simulink model "filtros_r2015b"  (R2015b)
settings: Solver=VariableStepAuto  SolverMode=SingleTasking  StartTime=0.0  StopTime=10.0  RelTol=1e-3
libraries: dsparch4 x4
(part 4 of 5)

== system filtros_r2015b/filtro_bs_iir_direct2_sos_40_fb ==
  In : Inport
  Input Quantizer : DataTypeConversion  OutDataTypeStr=fixdt(1,16,15)  RndMeth=Round  SaturateOnIntegerOverflow=on
  filter : dsparch4/Biquad Filter  FilterSource=Specify via dialog  CoeffSource=Specify via dialog  FilterObject=BQF  IIRFiltStruct=Direct form II  BiQuadCoeffs=[1 -1.11152954346655419 1.05088219447620013 1 -0.813428281179642165 0.552005579906472033;1 -1.07211536629555804 1.06865251897541036 1 -0.742197661664668717 0.854865767395351028;1 -1.0032399136855954 0.935758131903575485 1 -1.18020037227255226 0.875550994084790757;1 -1.01063368621325411 1.03083232416279569 1 -0.8635074436780521 0.959930995951585597;1 -1.05770999558857559 0.951581007807177359 1 -1.17581613832315401 0.964163580544992183;1 -0.980405596804986956 0.97009053687980229 1 -0.90563072038096426 0.990340187952881257;1 -1.1019651730511173 0.999999494703609493 1 -1.16875024700793517 0.991207917022611129]  ScaleValues=[0.619240669533610344;1;1;1;1;1;1;1]  IC=0  ICnum=0  ICden=0  a0Flag=Warning  optimizeScaleValues=on  ScaleValueMode=Specify via input port (g)  InputProcessing=Columns as channels (frame based)  roundingMode=Convergent  overflowMode=off  stageInputMode=Binary point scaling  stageInputWordLength=16  stageInputFracLength=10  stageOutputMode=Binary point scaling  stageOutputWordLength=16  stageOutputFracLength=11  firstCoeffMode=Binary point scaling  firstCoeffWordLength=40  firstCoeffFracLength=38  scaleValueFracLength=39  prodOutputMode=Binary point scaling  prodOutputWordLength=56  prodOutputFracLength=53  denProdOutputFracLength=53  accumMode=Binary point scaling  accumWordLength=40  accumFracLength=35  denAccumFracLength=35  memoryMode=Binary point scaling  memoryWordLength=16  memoryFracLength=15  secondMemoryFracLength=15  outputMode=Binary point scaling  outputWordLength=16  outputFracLength=11
  Out : Outport
  wires:
  In/1 -> Input Quantizer/1
  Input Quantizer/1 -> filter/1
  filter/1 -> Out/1

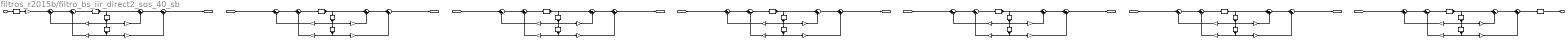
== system filtros_r2015b/filtro_bs_iir_direct2_sos_40_sb ==
  Input : Inport
  CastState{1..7} (7 alike) : DataTypeConversion  OutDataTypeStr=fixdt(1,16,15)  RndMeth=Convergent
  ConvertIn : DataTypeConversion  OutDataTypeStr=fixdt(1,16,15)  RndMeth=Nearest  SaturateOnIntegerOverflow=on
  ConvertOut : DataTypeConversion  OutDataTypeStr=fixdt(1,16,11)  RndMeth=Convergent
  Delay{11..17,21..27} (14 alike) : Delay  DelayLength=1  InitialCondition=0
  SumA{21..27,31..37} (14 alike) : Sum  Inputs=|+-  AccumDataTypeStr=fixdt(1,40,35)  OutDataTypeStr=fixdt(1,40,35)  RndMeth=Convergent
  SumB{21..27,31..37} (14 alike) : Sum  Inputs=|++  AccumDataTypeStr=fixdt(1,40,35)  OutDataTypeStr=fixdt(1,40,35)  RndMeth=Convergent
  a(2)(1) : Gain  Gain=-0.813428281179642165  ParamDataTypeStr=fixdt(1,40,38)  OutDataTypeStr=fixdt(1,56,53)  RndMeth=Convergent
  a(2)(2) : Gain  Gain=-0.742197661664668717  ParamDataTypeStr=fixdt(1,40,38)  OutDataTypeStr=fixdt(1,56,53)  RndMeth=Convergent
  a(2)(3) : Gain  Gain=-1.18020037227255226  ParamDataTypeStr=fixdt(1,40,38)  OutDataTypeStr=fixdt(1,56,53)  RndMeth=Convergent
  a(2)(4) : Gain  Gain=-0.8635074436780521  ParamDataTypeStr=fixdt(1,40,38)  OutDataTypeStr=fixdt(1,56,53)  RndMeth=Convergent
  a(2)(5) : Gain  Gain=-1.17581613832315401  ParamDataTypeStr=fixdt(1,40,38)  OutDataTypeStr=fixdt(1,56,53)  RndMeth=Convergent
  a(2)(6) : Gain  Gain=-0.90563072038096426  ParamDataTypeStr=fixdt(1,40,38)  OutDataTypeStr=fixdt(1,56,53)  RndMeth=Convergent
  a(2)(7) : Gain  Gain=-1.16875024700793517  ParamDataTypeStr=fixdt(1,40,38)  OutDataTypeStr=fixdt(1,56,53)  RndMeth=Convergent
  a(3)(1) : Gain  Gain=0.552005579906472033  ParamDataTypeStr=fixdt(1,40,38)  OutDataTypeStr=fixdt(1,56,53)  RndMeth=Convergent
  a(3)(2) : Gain  Gain=0.854865767395351028  ParamDataTypeStr=fixdt(1,40,38)  OutDataTypeStr=fixdt(1,56,53)  RndMeth=Convergent
  a(3)(3) : Gain  Gain=0.875550994084790757  ParamDataTypeStr=fixdt(1,40,38)  OutDataTypeStr=fixdt(1,56,53)  RndMeth=Convergent
  a(3)(4) : Gain  Gain=0.959930995951585597  ParamDataTypeStr=fixdt(1,40,38)  OutDataTypeStr=fixdt(1,56,53)  RndMeth=Convergent
  a(3)(5) : Gain  Gain=0.964163580544992183  ParamDataTypeStr=fixdt(1,40,38)  OutDataTypeStr=fixdt(1,56,53)  RndMeth=Convergent
  a(3)(6) : Gain  Gain=0.990340187952881257  ParamDataTypeStr=fixdt(1,40,38)  OutDataTypeStr=fixdt(1,56,53)  RndMeth=Convergent
  a(3)(7) : Gain  Gain=0.991207917022611129  ParamDataTypeStr=fixdt(1,40,38)  OutDataTypeStr=fixdt(1,56,53)  RndMeth=Convergent
  b(2)(1) : Gain  Gain=-1.11152954346655419  ParamDataTypeStr=fixdt(1,40,38)  OutDataTypeStr=fixdt(1,56,53)  RndMeth=Convergent
  b(2)(2) : Gain  Gain=-1.07211536629555804  ParamDataTypeStr=fixdt(1,40,38)  OutDataTypeStr=fixdt(1,56,53)  RndMeth=Convergent
  b(2)(3) : Gain  Gain=-1.0032399136855954  ParamDataTypeStr=fixdt(1,40,38)  OutDataTypeStr=fixdt(1,56,53)  RndMeth=Convergent
  b(2)(4) : Gain  Gain=-1.01063368621325411  ParamDataTypeStr=fixdt(1,40,38)  OutDataTypeStr=fixdt(1,56,53)  RndMeth=Convergent
  b(2)(5) : Gain  Gain=-1.05770999558857559  ParamDataTypeStr=fixdt(1,40,38)  OutDataTypeStr=fixdt(1,56,53)  RndMeth=Convergent
  b(2)(6) : Gain  Gain=-0.980405596804986956  ParamDataTypeStr=fixdt(1,40,38)  OutDataTypeStr=fixdt(1,56,53)  RndMeth=Convergent
  b(2)(7) : Gain  Gain=-1.1019651730511173  ParamDataTypeStr=fixdt(1,40,38)  OutDataTypeStr=fixdt(1,56,53)  RndMeth=Convergent
  b(3)(1) : Gain  Gain=1.05088219447620013  ParamDataTypeStr=fixdt(1,40,38)  OutDataTypeStr=fixdt(1,56,53)  RndMeth=Convergent
  b(3)(2) : Gain  Gain=1.06865251897541036  ParamDataTypeStr=fixdt(1,40,38)  OutDataTypeStr=fixdt(1,56,53)  RndMeth=Convergent
  b(3)(3) : Gain  Gain=0.935758131903575485  ParamDataTypeStr=fixdt(1,40,38)  OutDataTypeStr=fixdt(1,56,53)  RndMeth=Convergent
  b(3)(4) : Gain  Gain=1.03083232416279569  ParamDataTypeStr=fixdt(1,40,38)  OutDataTypeStr=fixdt(1,56,53)  RndMeth=Convergent
  b(3)(5) : Gain  Gain=0.951581007807177359  ParamDataTypeStr=fixdt(1,40,38)  OutDataTypeStr=fixdt(1,56,53)  RndMeth=Convergent
  b(3)(6) : Gain  Gain=0.97009053687980229  ParamDataTypeStr=fixdt(1,40,38)  OutDataTypeStr=fixdt(1,56,53)  RndMeth=Convergent
  b(3)(7) : Gain  Gain=0.999999494703609493  ParamDataTypeStr=fixdt(1,40,38)  OutDataTypeStr=fixdt(1,56,53)  RndMeth=Convergent
  s(1) : Gain  Gain=0.619240669533610344  ParamDataTypeStr=fixdt(1,40,39)  OutDataTypeStr=fixdt(1,16,10)  RndMeth=Convergent
  Output : Outport
  wires:
  Input/1 -> ConvertIn/1
  s(1)/1 -> SumA21/1
  SumA21/1 -> SumA31/1
  SumA31/1 -> CastState1/1
  CastState1/1 -> SumB21/1, Delay11/1
  SumB21/1 -> SumB31/1
  SumB31/1 -> [Sect1]
  a(2)(1)/1 -> SumA21/2
  Delay11/1 -> a(2)(1)/1, b(2)(1)/1, Delay21/1
  b(2)(1)/1 -> SumB21/2
  a(3)(1)/1 -> SumA31/2
  Delay21/1 -> a(3)(1)/1, b(3)(1)/1
  b(3)(1)/1 -> SumB31/2
  ConvertIn/1 -> s(1)/1
  [Sect1] -> SumA22/1
  SumA22/1 -> SumA32/1
  SumA32/1 -> CastState2/1
  CastState2/1 -> SumB22/1, Delay12/1
  SumB22/1 -> SumB32/1
  SumB32/1 -> [Sect2]
  a(2)(2)/1 -> SumA22/2
  Delay12/1 -> a(2)(2)/1, b(2)(2)/1, Delay22/1
  b(2)(2)/1 -> SumB22/2
  a(3)(2)/1 -> SumA32/2
  Delay22/1 -> a(3)(2)/1, b(3)(2)/1
  b(3)(2)/1 -> SumB32/2
  [Sect2] -> SumA23/1
  SumA23/1 -> SumA33/1
  SumA33/1 -> CastState3/1
  CastState3/1 -> SumB23/1, Delay13/1
  SumB23/1 -> SumB33/1
  SumB33/1 -> [Sect3]
  a(2)(3)/1 -> SumA23/2
  Delay13/1 -> a(2)(3)/1, b(2)(3)/1, Delay23/1
  b(2)(3)/1 -> SumB23/2
  a(3)(3)/1 -> SumA33/2
  Delay23/1 -> a(3)(3)/1, b(3)(3)/1
  b(3)(3)/1 -> SumB33/2
  [Sect3] -> SumA24/1
  SumA24/1 -> SumA34/1
  SumA34/1 -> CastState4/1
  CastState4/1 -> SumB24/1, Delay14/1
  SumB24/1 -> SumB34/1
  SumB34/1 -> [Sect4]
  a(2)(4)/1 -> SumA24/2
  Delay14/1 -> a(2)(4)/1, b(2)(4)/1, Delay24/1
  b(2)(4)/1 -> SumB24/2
  a(3)(4)/1 -> SumA34/2
  Delay24/1 -> a(3)(4)/1, b(3)(4)/1
  b(3)(4)/1 -> SumB34/2
  [Sect4] -> SumA25/1
  SumA25/1 -> SumA35/1
  SumA35/1 -> CastState5/1
  CastState5/1 -> SumB25/1, Delay15/1
  SumB25/1 -> SumB35/1
  SumB35/1 -> [Sect5]
  a(2)(5)/1 -> SumA25/2
  Delay15/1 -> a(2)(5)/1, b(2)(5)/1, Delay25/1
  b(2)(5)/1 -> SumB25/2
  a(3)(5)/1 -> SumA35/2
  Delay25/1 -> a(3)(5)/1, b(3)(5)/1
  b(3)(5)/1 -> SumB35/2
  [Sect5] -> SumA26/1
  SumA26/1 -> SumA36/1
  SumA36/1 -> CastState6/1
  CastState6/1 -> SumB26/1, Delay16/1
  SumB26/1 -> SumB36/1
  SumB36/1 -> [Sect6]
  a(2)(6)/1 -> SumA26/2
  Delay16/1 -> a(2)(6)/1, b(2)(6)/1, Delay26/1
  b(2)(6)/1 -> SumB26/2
  a(3)(6)/1 -> SumA36/2
  Delay26/1 -> a(3)(6)/1, b(3)(6)/1
  b(3)(6)/1 -> SumB36/2
  [Sect6] -> SumA27/1
  SumA27/1 -> SumA37/1
  SumA37/1 -> CastState7/1
  CastState7/1 -> SumB27/1, Delay17/1
  SumB27/1 -> SumB37/1
  SumB37/1 -> ConvertOut/1
  a(2)(7)/1 -> SumA27/2
  Delay17/1 -> a(2)(7)/1, b(2)(7)/1, Delay27/1
  b(2)(7)/1 -> SumB27/2
  a(3)(7)/1 -> SumA37/2
  Delay27/1 -> a(3)(7)/1, b(3)(7)/1
  b(3)(7)/1 -> SumB37/2
  ConvertOut/1 -> Output/1

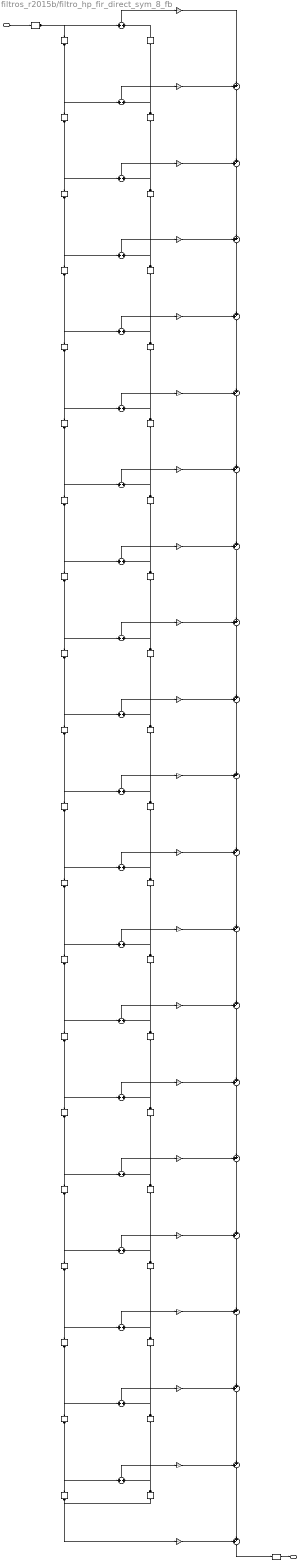
== system filtros_r2015b/filtro_hp_fir_direct_sym_8_fb ==
  Input : Inport
  BodyDelayL{2..20} (19 alike) : Delay  DelayLength=1  InitialCondition=0  InputProcessing=Columns as channels (frame based)
  BodyDelayR{2..20} (19 alike) : Delay  DelayLength=1  InitialCondition=0  InputProcessing=Columns as channels (frame based)
  BodySumL{2..20} (19 alike) : Sum  Inputs=+|+  AccumDataTypeStr=fixdt(1,17,15)  OutDataTypeStr=fixdt(1,17,15)  RndMeth=Convergent
  BodySumR{2..20} (19 alike) : Sum  Inputs=++|  AccumDataTypeStr=fixdt(1,26,24)  OutDataTypeStr=fixdt(1,26,24)  RndMeth=Convergent
  ConvertIn : DataTypeConversion  OutDataTypeStr=fixdt(1,16,15)  RndMeth=Nearest  SaturateOnIntegerOverflow=on
  ConvertOut : DataTypeConversion  OutDataTypeStr=fixdt(1,26,24)  RndMeth=Convergent
  FootDelayL21 : Delay  DelayLength=1  InitialCondition=0  InputProcessing=Columns as channels (frame based)
  FootSumR21 : Sum  Inputs=++|  AccumDataTypeStr=fixdt(1,26,24)  OutDataTypeStr=fixdt(1,26,24)  RndMeth=Convergent
  HeadDelayR1 : Delay  DelayLength=1  InitialCondition=0  InputProcessing=Columns as channels (frame based)
  HeadSumL1 : Sum  Inputs=+|+  AccumDataTypeStr=fixdt(1,17,15)  OutDataTypeStr=fixdt(1,17,15)  RndMeth=Convergent
  h(1) : Gain  Gain=0.00147457494090809035  ParamDataTypeStr=fixdt(1,9,9)  OutDataTypeStr=fixdt(1,25,24)  RndMeth=Convergent
  h(10) : Gain  Gain=-0.0215233057817383611  ParamDataTypeStr=fixdt(1,9,9)  OutDataTypeStr=fixdt(1,25,24)  RndMeth=Convergent
  h(11) : Gain  Gain=0.00302086608454419422  ParamDataTypeStr=fixdt(1,9,9)  OutDataTypeStr=fixdt(1,25,24)  RndMeth=Convergent
  h(12) : Gain  Gain=0.026471417892813251  ParamDataTypeStr=fixdt(1,9,9)  OutDataTypeStr=fixdt(1,25,24)  RndMeth=Convergent
  h(13) : Gain  Gain=-0.0223937353592350563  ParamDataTypeStr=fixdt(1,9,9)  OutDataTypeStr=fixdt(1,25,24)  RndMeth=Convergent
  h(14) : Gain  Gain=-0.0205814623315632092  ParamDataTypeStr=fixdt(1,9,9)  OutDataTypeStr=fixdt(1,25,24)  RndMeth=Convergent
  h(15) : Gain  Gain=0.04620278017582298  ParamDataTypeStr=fixdt(1,9,9)  OutDataTypeStr=fixdt(1,25,24)  RndMeth=Convergent
  h(16) : Gain  Gain=-0.00351180581067440717  ParamDataTypeStr=fixdt(1,9,9)  OutDataTypeStr=fixdt(1,25,24)  RndMeth=Convergent
  h(17) : Gain  Gain=-0.0693736142677181811  ParamDataTypeStr=fixdt(1,9,9)  OutDataTypeStr=fixdt(1,25,24)  RndMeth=Convergent
  h(18) : Gain  Gain=0.0618199572510256742  ParamDataTypeStr=fixdt(1,9,9)  OutDataTypeStr=fixdt(1,25,24)  RndMeth=Convergent
  h(19) : Gain  Gain=0.0862516021295114677  ParamDataTypeStr=fixdt(1,9,9)  OutDataTypeStr=fixdt(1,25,24)  RndMeth=Convergent
  h(2) : Gain  Gain=0.00619384132880984074  ParamDataTypeStr=fixdt(1,9,9)  OutDataTypeStr=fixdt(1,25,24)  RndMeth=Convergent
  h(20) : Gain  Gain=-0.291540360141503418  ParamDataTypeStr=fixdt(1,9,9)  OutDataTypeStr=fixdt(1,25,24)  RndMeth=Convergent
  h(21) : Gain  Gain=0.388153726976887825  ParamDataTypeStr=fixdt(1,9,9)  OutDataTypeStr=fixdt(1,25,24)  RndMeth=Convergent
  h(3) : Gain  Gain=-0.00628903216358678557  ParamDataTypeStr=fixdt(1,9,9)  OutDataTypeStr=fixdt(1,25,24)  RndMeth=Convergent
  h(4) : Gain  Gain=-0.00399100484830938393  ParamDataTypeStr=fixdt(1,9,9)  OutDataTypeStr=fixdt(1,25,24)  RndMeth=Convergent
  h(5) : Gain  Gain=0.0110850821887358182  ParamDataTypeStr=fixdt(1,9,9)  OutDataTypeStr=fixdt(1,25,24)  RndMeth=Convergent
  h(6) : Gain  Gain=-0.00230036500462132672  ParamDataTypeStr=fixdt(1,9,9)  OutDataTypeStr=fixdt(1,25,24)  RndMeth=Convergent
  h(7) : Gain  Gain=-0.012964596819967358  ParamDataTypeStr=fixdt(1,9,9)  OutDataTypeStr=fixdt(1,25,24)  RndMeth=Convergent
  h(8) : Gain  Gain=0.011820806710017737  ParamDataTypeStr=fixdt(1,9,9)  OutDataTypeStr=fixdt(1,25,24)  RndMeth=Convergent
  h(9) : Gain  Gain=0.00889040068107843987  ParamDataTypeStr=fixdt(1,9,9)  OutDataTypeStr=fixdt(1,25,24)  RndMeth=Convergent
  Output : Outport
  wires:
  Input/1 -> ConvertIn/1
  HeadSumL1/1 -> h(1)/1
  h(1)/1 -> BodySumR2/2
  HeadDelayR1/1 -> HeadSumL1/2
  ConvertIn/1 -> HeadSumL1/1, BodyDelayL2/1
  BodyDelayL2/1 -> BodySumL2/1, BodyDelayL3/1
  BodySumL2/1 -> h(2)/1
  h(2)/1 -> BodySumR2/1
  BodyDelayR2/1 -> BodySumL2/2, HeadDelayR1/1
  BodySumR2/1 -> BodySumR3/2
  BodyDelayL3/1 -> BodySumL3/1, BodyDelayL4/1
  BodySumL3/1 -> h(3)/1
  h(3)/1 -> BodySumR3/1
  BodyDelayR3/1 -> BodySumL3/2, BodyDelayR2/1
  BodySumR3/1 -> BodySumR4/2
  BodyDelayL4/1 -> BodySumL4/1, BodyDelayL5/1
  BodySumL4/1 -> h(4)/1
  h(4)/1 -> BodySumR4/1
  BodyDelayR4/1 -> BodySumL4/2, BodyDelayR3/1
  BodySumR4/1 -> BodySumR5/2
  BodyDelayL5/1 -> BodySumL5/1, BodyDelayL6/1
  BodySumL5/1 -> h(5)/1
  h(5)/1 -> BodySumR5/1
  BodyDelayR5/1 -> BodySumL5/2, BodyDelayR4/1
  BodySumR5/1 -> BodySumR6/2
  BodyDelayL6/1 -> BodySumL6/1, BodyDelayL7/1
  BodySumL6/1 -> h(6)/1
  h(6)/1 -> BodySumR6/1
  BodyDelayR6/1 -> BodySumL6/2, BodyDelayR5/1
  BodySumR6/1 -> BodySumR7/2
  BodyDelayL7/1 -> BodySumL7/1, BodyDelayL8/1
  BodySumL7/1 -> h(7)/1
  h(7)/1 -> BodySumR7/1
  BodyDelayR7/1 -> BodySumL7/2, BodyDelayR6/1
  BodySumR7/1 -> BodySumR8/2
  BodyDelayL8/1 -> BodySumL8/1, BodyDelayL9/1
  BodySumL8/1 -> h(8)/1
  h(8)/1 -> BodySumR8/1
  BodyDelayR8/1 -> BodySumL8/2, BodyDelayR7/1
  BodySumR8/1 -> BodySumR9/2
  BodyDelayL9/1 -> BodySumL9/1, BodyDelayL10/1
  BodySumL9/1 -> h(9)/1
  h(9)/1 -> BodySumR9/1
  BodyDelayR9/1 -> BodySumL9/2, BodyDelayR8/1
  BodySumR9/1 -> BodySumR10/2
  BodyDelayL10/1 -> BodySumL10/1, BodyDelayL11/1
  BodySumL10/1 -> h(10)/1
  h(10)/1 -> BodySumR10/1
  BodyDelayR10/1 -> BodySumL10/2, BodyDelayR9/1
  BodySumR10/1 -> BodySumR11/2
  BodyDelayL11/1 -> BodySumL11/1, BodyDelayL12/1
  BodySumL11/1 -> h(11)/1
  h(11)/1 -> BodySumR11/1
  BodyDelayR11/1 -> BodySumL11/2, BodyDelayR10/1
  BodySumR11/1 -> BodySumR12/2
  BodyDelayL12/1 -> BodySumL12/1, BodyDelayL13/1
  BodySumL12/1 -> h(12)/1
  h(12)/1 -> BodySumR12/1
  BodyDelayR12/1 -> BodySumL12/2, BodyDelayR11/1
  BodySumR12/1 -> BodySumR13/2
  BodyDelayL13/1 -> BodySumL13/1, BodyDelayL14/1
  BodySumL13/1 -> h(13)/1
  h(13)/1 -> BodySumR13/1
  BodyDelayR13/1 -> BodySumL13/2, BodyDelayR12/1
  BodySumR13/1 -> BodySumR14/2
  BodyDelayL14/1 -> BodySumL14/1, BodyDelayL15/1
  BodySumL14/1 -> h(14)/1
  h(14)/1 -> BodySumR14/1
  BodyDelayR14/1 -> BodySumL14/2, BodyDelayR13/1
  BodySumR14/1 -> BodySumR15/2
  BodyDelayL15/1 -> BodySumL15/1, BodyDelayL16/1
  BodySumL15/1 -> h(15)/1
  h(15)/1 -> BodySumR15/1
  BodyDelayR15/1 -> BodySumL15/2, BodyDelayR14/1
  BodySumR15/1 -> BodySumR16/2
  BodyDelayL16/1 -> BodySumL16/1, BodyDelayL17/1
  BodySumL16/1 -> h(16)/1
  h(16)/1 -> BodySumR16/1
  BodyDelayR16/1 -> BodySumL16/2, BodyDelayR15/1
  BodySumR16/1 -> BodySumR17/2
  BodyDelayL17/1 -> BodySumL17/1, BodyDelayL18/1
  BodySumL17/1 -> h(17)/1
  h(17)/1 -> BodySumR17/1
  BodyDelayR17/1 -> BodySumL17/2, BodyDelayR16/1
  BodySumR17/1 -> BodySumR18/2
  BodyDelayL18/1 -> BodySumL18/1, BodyDelayL19/1
  BodySumL18/1 -> h(18)/1
  h(18)/1 -> BodySumR18/1
  BodyDelayR18/1 -> BodySumL18/2, BodyDelayR17/1
  BodySumR18/1 -> BodySumR19/2
  BodyDelayL19/1 -> BodySumL19/1, BodyDelayL20/1
  BodySumL19/1 -> h(19)/1
  h(19)/1 -> BodySumR19/1
  BodyDelayR19/1 -> BodySumL19/2, BodyDelayR18/1
  BodySumR19/1 -> BodySumR20/2
  BodyDelayL20/1 -> BodySumL20/1, FootDelayL21/1
  BodySumL20/1 -> h(20)/1
  h(20)/1 -> BodySumR20/1
  BodyDelayR20/1 -> BodySumL20/2, BodyDelayR19/1
  BodySumR20/1 -> FootSumR21/2
  FootDelayL21/1 -> h(21)/1, BodyDelayR20/1
  h(21)/1 -> FootSumR21/1
  FootSumR21/1 -> ConvertOut/1
  ConvertOut/1 -> Output/1

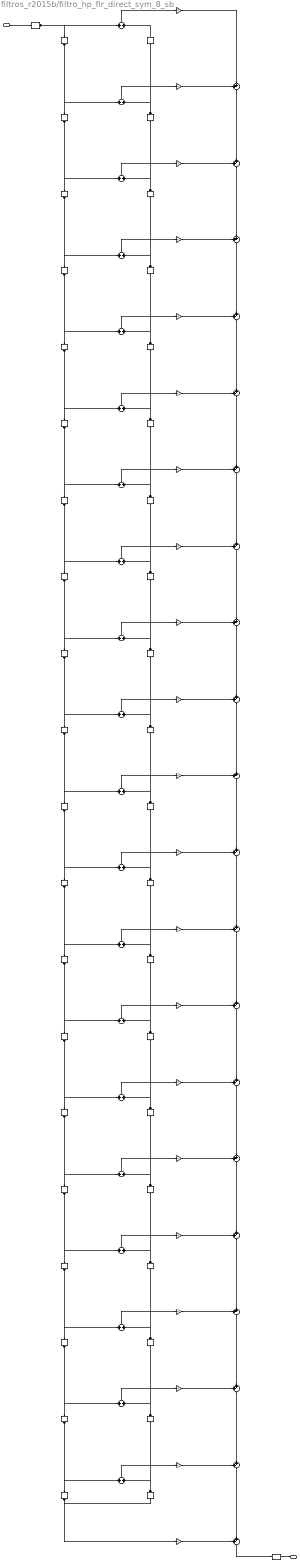
== system filtros_r2015b/filtro_hp_fir_direct_sym_8_sb ==
  Input : Inport
  BodyDelayL{2..20} (19 alike) : Delay  DelayLength=1  InitialCondition=0
  BodyDelayR{2..20} (19 alike) : Delay  DelayLength=1  InitialCondition=0
  BodySumL{2..20} (19 alike) : Sum  Inputs=+|+  AccumDataTypeStr=fixdt(1,17,15)  OutDataTypeStr=fixdt(1,17,15)  RndMeth=Convergent
  BodySumR{2..20} (19 alike) : Sum  Inputs=++|  AccumDataTypeStr=fixdt(1,26,24)  OutDataTypeStr=fixdt(1,26,24)  RndMeth=Convergent
  ConvertIn : DataTypeConversion  OutDataTypeStr=fixdt(1,16,15)  RndMeth=Nearest  SaturateOnIntegerOverflow=on
  ConvertOut : DataTypeConversion  OutDataTypeStr=fixdt(1,26,24)  RndMeth=Convergent
  FootDelayL21 : Delay  DelayLength=1  InitialCondition=0
  FootSumR21 : Sum  Inputs=++|  AccumDataTypeStr=fixdt(1,26,24)  OutDataTypeStr=fixdt(1,26,24)  RndMeth=Convergent
  HeadDelayR1 : Delay  DelayLength=1  InitialCondition=0
  HeadSumL1 : Sum  Inputs=+|+  AccumDataTypeStr=fixdt(1,17,15)  OutDataTypeStr=fixdt(1,17,15)  RndMeth=Convergent
  h(1) : Gain  Gain=0.00147457494090809035  ParamDataTypeStr=fixdt(1,9,9)  OutDataTypeStr=fixdt(1,25,24)  RndMeth=Convergent
  h(10) : Gain  Gain=-0.0215233057817383611  ParamDataTypeStr=fixdt(1,9,9)  OutDataTypeStr=fixdt(1,25,24)  RndMeth=Convergent
  h(11) : Gain  Gain=0.00302086608454419422  ParamDataTypeStr=fixdt(1,9,9)  OutDataTypeStr=fixdt(1,25,24)  RndMeth=Convergent
  h(12) : Gain  Gain=0.026471417892813251  ParamDataTypeStr=fixdt(1,9,9)  OutDataTypeStr=fixdt(1,25,24)  RndMeth=Convergent
  h(13) : Gain  Gain=-0.0223937353592350563  ParamDataTypeStr=fixdt(1,9,9)  OutDataTypeStr=fixdt(1,25,24)  RndMeth=Convergent
  h(14) : Gain  Gain=-0.0205814623315632092  ParamDataTypeStr=fixdt(1,9,9)  OutDataTypeStr=fixdt(1,25,24)  RndMeth=Convergent
  h(15) : Gain  Gain=0.04620278017582298  ParamDataTypeStr=fixdt(1,9,9)  OutDataTypeStr=fixdt(1,25,24)  RndMeth=Convergent
  h(16) : Gain  Gain=-0.00351180581067440717  ParamDataTypeStr=fixdt(1,9,9)  OutDataTypeStr=fixdt(1,25,24)  RndMeth=Convergent
  h(17) : Gain  Gain=-0.0693736142677181811  ParamDataTypeStr=fixdt(1,9,9)  OutDataTypeStr=fixdt(1,25,24)  RndMeth=Convergent
  h(18) : Gain  Gain=0.0618199572510256742  ParamDataTypeStr=fixdt(1,9,9)  OutDataTypeStr=fixdt(1,25,24)  RndMeth=Convergent
  h(19) : Gain  Gain=0.0862516021295114677  ParamDataTypeStr=fixdt(1,9,9)  OutDataTypeStr=fixdt(1,25,24)  RndMeth=Convergent
  h(2) : Gain  Gain=0.00619384132880984074  ParamDataTypeStr=fixdt(1,9,9)  OutDataTypeStr=fixdt(1,25,24)  RndMeth=Convergent
  h(20) : Gain  Gain=-0.291540360141503418  ParamDataTypeStr=fixdt(1,9,9)  OutDataTypeStr=fixdt(1,25,24)  RndMeth=Convergent
  h(21) : Gain  Gain=0.388153726976887825  ParamDataTypeStr=fixdt(1,9,9)  OutDataTypeStr=fixdt(1,25,24)  RndMeth=Convergent
  h(3) : Gain  Gain=-0.00628903216358678557  ParamDataTypeStr=fixdt(1,9,9)  OutDataTypeStr=fixdt(1,25,24)  RndMeth=Convergent
  h(4) : Gain  Gain=-0.00399100484830938393  ParamDataTypeStr=fixdt(1,9,9)  OutDataTypeStr=fixdt(1,25,24)  RndMeth=Convergent
  h(5) : Gain  Gain=0.0110850821887358182  ParamDataTypeStr=fixdt(1,9,9)  OutDataTypeStr=fixdt(1,25,24)  RndMeth=Convergent
  h(6) : Gain  Gain=-0.00230036500462132672  ParamDataTypeStr=fixdt(1,9,9)  OutDataTypeStr=fixdt(1,25,24)  RndMeth=Convergent
  h(7) : Gain  Gain=-0.012964596819967358  ParamDataTypeStr=fixdt(1,9,9)  OutDataTypeStr=fixdt(1,25,24)  RndMeth=Convergent
  h(8) : Gain  Gain=0.011820806710017737  ParamDataTypeStr=fixdt(1,9,9)  OutDataTypeStr=fixdt(1,25,24)  RndMeth=Convergent
  h(9) : Gain  Gain=0.00889040068107843987  ParamDataTypeStr=fixdt(1,9,9)  OutDataTypeStr=fixdt(1,25,24)  RndMeth=Convergent
  Output : Outport
  wires:
  Input/1 -> ConvertIn/1
  HeadSumL1/1 -> h(1)/1
  h(1)/1 -> BodySumR2/2
  HeadDelayR1/1 -> HeadSumL1/2
  ConvertIn/1 -> HeadSumL1/1, BodyDelayL2/1
  BodyDelayL2/1 -> BodySumL2/1, BodyDelayL3/1
  BodySumL2/1 -> h(2)/1
  h(2)/1 -> BodySumR2/1
  BodyDelayR2/1 -> BodySumL2/2, HeadDelayR1/1
  BodySumR2/1 -> BodySumR3/2
  BodyDelayL3/1 -> BodySumL3/1, BodyDelayL4/1
  BodySumL3/1 -> h(3)/1
  h(3)/1 -> BodySumR3/1
  BodyDelayR3/1 -> BodySumL3/2, BodyDelayR2/1
  BodySumR3/1 -> BodySumR4/2
  BodyDelayL4/1 -> BodySumL4/1, BodyDelayL5/1
  BodySumL4/1 -> h(4)/1
  h(4)/1 -> BodySumR4/1
  BodyDelayR4/1 -> BodySumL4/2, BodyDelayR3/1
  BodySumR4/1 -> BodySumR5/2
  BodyDelayL5/1 -> BodySumL5/1, BodyDelayL6/1
  BodySumL5/1 -> h(5)/1
  h(5)/1 -> BodySumR5/1
  BodyDelayR5/1 -> BodySumL5/2, BodyDelayR4/1
  BodySumR5/1 -> BodySumR6/2
  BodyDelayL6/1 -> BodySumL6/1, BodyDelayL7/1
  BodySumL6/1 -> h(6)/1
  h(6)/1 -> BodySumR6/1
  BodyDelayR6/1 -> BodySumL6/2, BodyDelayR5/1
  BodySumR6/1 -> BodySumR7/2
  BodyDelayL7/1 -> BodySumL7/1, BodyDelayL8/1
  BodySumL7/1 -> h(7)/1
  h(7)/1 -> BodySumR7/1
  BodyDelayR7/1 -> BodySumL7/2, BodyDelayR6/1
  BodySumR7/1 -> BodySumR8/2
  BodyDelayL8/1 -> BodySumL8/1, BodyDelayL9/1
  BodySumL8/1 -> h(8)/1
  h(8)/1 -> BodySumR8/1
  BodyDelayR8/1 -> BodySumL8/2, BodyDelayR7/1
  BodySumR8/1 -> BodySumR9/2
  BodyDelayL9/1 -> BodySumL9/1, BodyDelayL10/1
  BodySumL9/1 -> h(9)/1
  h(9)/1 -> BodySumR9/1
  BodyDelayR9/1 -> BodySumL9/2, BodyDelayR8/1
  BodySumR9/1 -> BodySumR10/2
  BodyDelayL10/1 -> BodySumL10/1, BodyDelayL11/1
  BodySumL10/1 -> h(10)/1
  h(10)/1 -> BodySumR10/1
  BodyDelayR10/1 -> BodySumL10/2, BodyDelayR9/1
  BodySumR10/1 -> BodySumR11/2
  BodyDelayL11/1 -> BodySumL11/1, BodyDelayL12/1
  BodySumL11/1 -> h(11)/1
  h(11)/1 -> BodySumR11/1
  BodyDelayR11/1 -> BodySumL11/2, BodyDelayR10/1
  BodySumR11/1 -> BodySumR12/2
  BodyDelayL12/1 -> BodySumL12/1, BodyDelayL13/1
  BodySumL12/1 -> h(12)/1
  h(12)/1 -> BodySumR12/1
  BodyDelayR12/1 -> BodySumL12/2, BodyDelayR11/1
  BodySumR12/1 -> BodySumR13/2
  BodyDelayL13/1 -> BodySumL13/1, BodyDelayL14/1
  BodySumL13/1 -> h(13)/1
  h(13)/1 -> BodySumR13/1
  BodyDelayR13/1 -> BodySumL13/2, BodyDelayR12/1
  BodySumR13/1 -> BodySumR14/2
  BodyDelayL14/1 -> BodySumL14/1, BodyDelayL15/1
  BodySumL14/1 -> h(14)/1
  h(14)/1 -> BodySumR14/1
  BodyDelayR14/1 -> BodySumL14/2, BodyDelayR13/1
  BodySumR14/1 -> BodySumR15/2
  BodyDelayL15/1 -> BodySumL15/1, BodyDelayL16/1
  BodySumL15/1 -> h(15)/1
  h(15)/1 -> BodySumR15/1
  BodyDelayR15/1 -> BodySumL15/2, BodyDelayR14/1
  BodySumR15/1 -> BodySumR16/2
  BodyDelayL16/1 -> BodySumL16/1, BodyDelayL17/1
  BodySumL16/1 -> h(16)/1
  h(16)/1 -> BodySumR16/1
  BodyDelayR16/1 -> BodySumL16/2, BodyDelayR15/1
  BodySumR16/1 -> BodySumR17/2
  BodyDelayL17/1 -> BodySumL17/1, BodyDelayL18/1
  BodySumL17/1 -> h(17)/1
  h(17)/1 -> BodySumR17/1
  BodyDelayR17/1 -> BodySumL17/2, BodyDelayR16/1
  BodySumR17/1 -> BodySumR18/2
  BodyDelayL18/1 -> BodySumL18/1, BodyDelayL19/1
  BodySumL18/1 -> h(18)/1
  h(18)/1 -> BodySumR18/1
  BodyDelayR18/1 -> BodySumL18/2, BodyDelayR17/1
  BodySumR18/1 -> BodySumR19/2
  BodyDelayL19/1 -> BodySumL19/1, BodyDelayL20/1
  BodySumL19/1 -> h(19)/1
  h(19)/1 -> BodySumR19/1
  BodyDelayR19/1 -> BodySumL19/2, BodyDelayR18/1
  BodySumR19/1 -> BodySumR20/2
  BodyDelayL20/1 -> BodySumL20/1, FootDelayL21/1
  BodySumL20/1 -> h(20)/1
  h(20)/1 -> BodySumR20/1
  BodyDelayR20/1 -> BodySumL20/2, BodyDelayR19/1
  BodySumR20/1 -> FootSumR21/2
  FootDelayL21/1 -> h(21)/1, BodyDelayR20/1
  h(21)/1 -> FootSumR21/1
  FootSumR21/1 -> ConvertOut/1
  ConvertOut/1 -> Output/1

== system filtros_r2015b/filtro_hp_iir_direct2_sos_12_fb ==
  In : Inport
  Input Quantizer : DataTypeConversion  OutDataTypeStr=fixdt(1,16,15)  RndMeth=Round  SaturateOnIntegerOverflow=on
  filter : dsparch4/Biquad Filter  FilterSource=Specify via dialog  CoeffSource=Specify via dialog  FilterObject=BQF  IIRFiltStruct=Direct form II  BiQuadCoeffs=[1 -0.99999999999989253 0 1 0.415474721603748653 0;1 -8.07609406410542263 19.479965706920094 1 0 0;1 -1.53376334450087937 3.35686333262635195 1 -0.0534464222346326817 0.155789387270914625;1 -1.6085731579110969 1.00000000000014611 1 0.912430013497696479 0.311516679849097922;1 -0.414584614039461674 0.0513347926297817794 1 0.700912460681827776 0.455486580885583192;1 -0.910081099356177647 0.999999999999969691 1 0.336705133533832024 0.516670640463280928;1 -0.456903720087069476 0.297897144122819202 1 0.672299092917526986 0.823202885567432596]  ScaleValues=[3.0517578125e-05;1;1;1;1;1;1;1]  IC=0  ICnum=0  ICden=0  a0Flag=Warning  optimizeScaleValues=on  ScaleValueMode=Specify via input port (g)  InputProcessing=Columns as channels (frame based)  roundingMode=Convergent  overflowMode=off  stageInputMode=Binary point scaling  stageInputWordLength=16  stageInputFracLength=20  stageOutputMode=Binary point scaling  stageOutputWordLength=16  stageOutputFracLength=7  firstCoeffMode=Binary point scaling  firstCoeffWordLength=12  firstCoeffFracLength=6  scaleValueFracLength=25  prodOutputMode=Binary point scaling  prodOutputWordLength=28  prodOutputFracLength=21  denProdOutputFracLength=25  accumMode=Binary point scaling  accumWordLength=30  accumFracLength=21  denAccumFracLength=25  memoryMode=Binary point scaling  memoryWordLength=16  memoryFracLength=15  secondMemoryFracLength=15  outputMode=Binary point scaling  outputWordLength=16  outputFracLength=7
  Out : Outport
  wires:
  In/1 -> Input Quantizer/1
  Input Quantizer/1 -> filter/1
  filter/1 -> Out/1

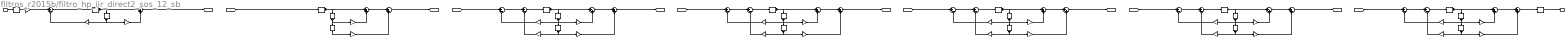
== system filtros_r2015b/filtro_hp_iir_direct2_sos_12_sb ==
  Input : Inport
  CastState{1..7} (7 alike) : DataTypeConversion  OutDataTypeStr=fixdt(1,16,15)  RndMeth=Convergent
  ConvertIn : DataTypeConversion  OutDataTypeStr=fixdt(1,16,15)  RndMeth=Nearest  SaturateOnIntegerOverflow=on
  ConvertOut : DataTypeConversion  OutDataTypeStr=fixdt(1,16,7)  RndMeth=Convergent
  Delay{11..17,22..27} (13 alike) : Delay  DelayLength=1  InitialCondition=0
  SumA{21,23..27,33..37} (11 alike) : Sum  Inputs=|+-  AccumDataTypeStr=fixdt(1,30,25)  OutDataTypeStr=fixdt(1,30,25)  RndMeth=Convergent
  SumB{21..27,32..37} (13 alike) : Sum  Inputs=|++  AccumDataTypeStr=fixdt(1,30,21)  OutDataTypeStr=fixdt(1,30,21)  RndMeth=Convergent
  a(2)(1) : Gain  Gain=0.415474721603748653  ParamDataTypeStr=fixdt(1,12,10)  OutDataTypeStr=fixdt(1,28,25)  RndMeth=Convergent
  a(2)(3) : Gain  Gain=-0.0534464222346326817  ParamDataTypeStr=fixdt(1,12,10)  OutDataTypeStr=fixdt(1,28,25)  RndMeth=Convergent
  a(2)(4) : Gain  Gain=0.912430013497696479  ParamDataTypeStr=fixdt(1,12,10)  OutDataTypeStr=fixdt(1,28,25)  RndMeth=Convergent
  a(2)(5) : Gain  Gain=0.700912460681827776  ParamDataTypeStr=fixdt(1,12,10)  OutDataTypeStr=fixdt(1,28,25)  RndMeth=Convergent
  a(2)(6) : Gain  Gain=0.336705133533832024  ParamDataTypeStr=fixdt(1,12,10)  OutDataTypeStr=fixdt(1,28,25)  RndMeth=Convergent
  a(2)(7) : Gain  Gain=0.672299092917526986  ParamDataTypeStr=fixdt(1,12,10)  OutDataTypeStr=fixdt(1,28,25)  RndMeth=Convergent
  a(3)(3) : Gain  Gain=0.155789387270914625  ParamDataTypeStr=fixdt(1,12,10)  OutDataTypeStr=fixdt(1,28,25)  RndMeth=Convergent
  a(3)(4) : Gain  Gain=0.311516679849097922  ParamDataTypeStr=fixdt(1,12,10)  OutDataTypeStr=fixdt(1,28,25)  RndMeth=Convergent
  a(3)(5) : Gain  Gain=0.455486580885583192  ParamDataTypeStr=fixdt(1,12,10)  OutDataTypeStr=fixdt(1,28,25)  RndMeth=Convergent
  a(3)(6) : Gain  Gain=0.516670640463280928  ParamDataTypeStr=fixdt(1,12,10)  OutDataTypeStr=fixdt(1,28,25)  RndMeth=Convergent
  a(3)(7) : Gain  Gain=0.823202885567432596  ParamDataTypeStr=fixdt(1,12,10)  OutDataTypeStr=fixdt(1,28,25)  RndMeth=Convergent
  b(2)(1) : Gain  Gain=-0.99999999999989253  ParamDataTypeStr=fixdt(1,12,6)  OutDataTypeStr=fixdt(1,28,21)  RndMeth=Convergent
  b(2)(2) : Gain  Gain=-8.07609406410542263  ParamDataTypeStr=fixdt(1,12,6)  OutDataTypeStr=fixdt(1,28,21)  RndMeth=Convergent
  b(2)(3) : Gain  Gain=-1.53376334450087937  ParamDataTypeStr=fixdt(1,12,6)  OutDataTypeStr=fixdt(1,28,21)  RndMeth=Convergent
  b(2)(4) : Gain  Gain=-1.6085731579110969  ParamDataTypeStr=fixdt(1,12,6)  OutDataTypeStr=fixdt(1,28,21)  RndMeth=Convergent
  b(2)(5) : Gain  Gain=-0.414584614039461674  ParamDataTypeStr=fixdt(1,12,6)  OutDataTypeStr=fixdt(1,28,21)  RndMeth=Convergent
  b(2)(6) : Gain  Gain=-0.910081099356177647  ParamDataTypeStr=fixdt(1,12,6)  OutDataTypeStr=fixdt(1,28,21)  RndMeth=Convergent
  b(2)(7) : Gain  Gain=-0.456903720087069476  ParamDataTypeStr=fixdt(1,12,6)  OutDataTypeStr=fixdt(1,28,21)  RndMeth=Convergent
  b(3)(2) : Gain  Gain=19.479965706920094  ParamDataTypeStr=fixdt(1,12,6)  OutDataTypeStr=fixdt(1,28,21)  RndMeth=Convergent
  b(3)(3) : Gain  Gain=3.35686333262635195  ParamDataTypeStr=fixdt(1,12,6)  OutDataTypeStr=fixdt(1,28,21)  RndMeth=Convergent
  b(3)(4) : Gain  Gain=1.00000000000014611  ParamDataTypeStr=fixdt(1,12,6)  OutDataTypeStr=fixdt(1,28,21)  RndMeth=Convergent
  b(3)(5) : Gain  Gain=0.0513347926297817794  ParamDataTypeStr=fixdt(1,12,6)  OutDataTypeStr=fixdt(1,28,21)  RndMeth=Convergent
  b(3)(6) : Gain  Gain=0.999999999999969691  ParamDataTypeStr=fixdt(1,12,6)  OutDataTypeStr=fixdt(1,28,21)  RndMeth=Convergent
  b(3)(7) : Gain  Gain=0.297897144122819202  ParamDataTypeStr=fixdt(1,12,6)  OutDataTypeStr=fixdt(1,28,21)  RndMeth=Convergent
  s(1) : Gain  Gain=3.0517578125e-05  ParamDataTypeStr=fixdt(1,12,25)  OutDataTypeStr=fixdt(1,16,20)  RndMeth=Convergent
  Output : Outport
  wires:
  Input/1 -> ConvertIn/1
  s(1)/1 -> SumA21/1
  SumA21/1 -> CastState1/1
  CastState1/1 -> SumB21/1, Delay11/1
  SumB21/1 -> [Sect1]
  a(2)(1)/1 -> SumA21/2
  Delay11/1 -> a(2)(1)/1, b(2)(1)/1
  b(2)(1)/1 -> SumB21/2
  ConvertIn/1 -> s(1)/1
  [Sect1] -> CastState2/1
  CastState2/1 -> SumB22/1, Delay12/1
  SumB22/1 -> SumB32/1
  SumB32/1 -> [Sect2]
  Delay12/1 -> b(2)(2)/1, Delay22/1
  b(2)(2)/1 -> SumB22/2
  Delay22/1 -> b(3)(2)/1
  b(3)(2)/1 -> SumB32/2
  [Sect2] -> SumA23/1
  SumA23/1 -> SumA33/1
  SumA33/1 -> CastState3/1
  CastState3/1 -> SumB23/1, Delay13/1
  SumB23/1 -> SumB33/1
  SumB33/1 -> [Sect3]
  a(2)(3)/1 -> SumA23/2
  Delay13/1 -> a(2)(3)/1, b(2)(3)/1, Delay23/1
  b(2)(3)/1 -> SumB23/2
  a(3)(3)/1 -> SumA33/2
  Delay23/1 -> a(3)(3)/1, b(3)(3)/1
  b(3)(3)/1 -> SumB33/2
  [Sect3] -> SumA24/1
  SumA24/1 -> SumA34/1
  SumA34/1 -> CastState4/1
  CastState4/1 -> SumB24/1, Delay14/1
  SumB24/1 -> SumB34/1
  SumB34/1 -> [Sect4]
  a(2)(4)/1 -> SumA24/2
  Delay14/1 -> a(2)(4)/1, b(2)(4)/1, Delay24/1
  b(2)(4)/1 -> SumB24/2
  a(3)(4)/1 -> SumA34/2
  Delay24/1 -> a(3)(4)/1, b(3)(4)/1
  b(3)(4)/1 -> SumB34/2
  [Sect4] -> SumA25/1
  SumA25/1 -> SumA35/1
  SumA35/1 -> CastState5/1
  CastState5/1 -> SumB25/1, Delay15/1
  SumB25/1 -> SumB35/1
  SumB35/1 -> [Sect5]
  a(2)(5)/1 -> SumA25/2
  Delay15/1 -> a(2)(5)/1, b(2)(5)/1, Delay25/1
  b(2)(5)/1 -> SumB25/2
  a(3)(5)/1 -> SumA35/2
  Delay25/1 -> a(3)(5)/1, b(3)(5)/1
  b(3)(5)/1 -> SumB35/2
  [Sect5] -> SumA26/1
  SumA26/1 -> SumA36/1
  SumA36/1 -> CastState6/1
  CastState6/1 -> SumB26/1, Delay16/1
  SumB26/1 -> SumB36/1
  SumB36/1 -> [Sect6]
  a(2)(6)/1 -> SumA26/2
  Delay16/1 -> a(2)(6)/1, b(2)(6)/1, Delay26/1
  b(2)(6)/1 -> SumB26/2
  a(3)(6)/1 -> SumA36/2
  Delay26/1 -> a(3)(6)/1, b(3)(6)/1
  b(3)(6)/1 -> SumB36/2
  [Sect6] -> SumA27/1
  SumA27/1 -> SumA37/1
  SumA37/1 -> CastState7/1
  CastState7/1 -> SumB27/1, Delay17/1
  SumB27/1 -> SumB37/1
  SumB37/1 -> ConvertOut/1
  a(2)(7)/1 -> SumA27/2
  Delay17/1 -> a(2)(7)/1, b(2)(7)/1, Delay27/1
  b(2)(7)/1 -> SumB27/2
  a(3)(7)/1 -> SumA37/2
  Delay27/1 -> a(3)(7)/1, b(3)(7)/1
  b(3)(7)/1 -> SumB37/2
  ConvertOut/1 -> Output/1

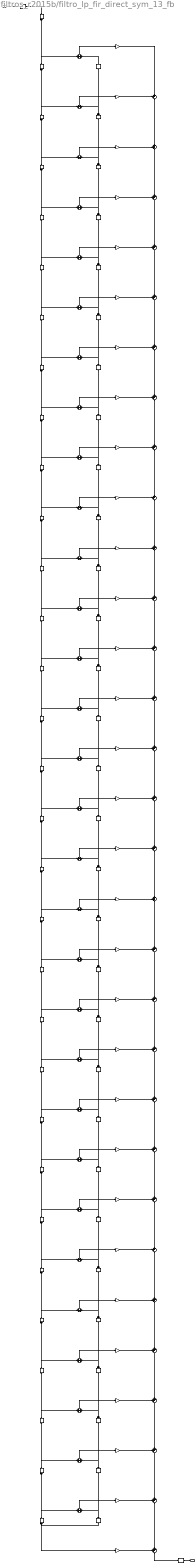
== system filtros_r2015b/filtro_lp_fir_direct_sym_13_fb ==
  Input : Inport
  BodyDelayL{2..31} (30 alike) : Delay  DelayLength=1  InitialCondition=0  InputProcessing=Columns as channels (frame based)
  BodyDelayR{2..31} (30 alike) : Delay  DelayLength=1  InitialCondition=0  InputProcessing=Columns as channels (frame based)
  BodySumL{2..31} (30 alike) : Sum  Inputs=+|+  AccumDataTypeStr=fixdt(1,17,15)  OutDataTypeStr=fixdt(1,17,15)  RndMeth=Convergent
  BodySumR{3..31} (29 alike) : Sum  Inputs=++|  AccumDataTypeStr=fixdt(1,30,27)  OutDataTypeStr=fixdt(1,30,27)  RndMeth=Convergent
  ConvertIn : DataTypeConversion  OutDataTypeStr=fixdt(1,16,15)  RndMeth=Nearest  SaturateOnIntegerOverflow=on
  ConvertOut : DataTypeConversion  OutDataTypeStr=fixdt(1,30,27)  RndMeth=Convergent
  FootDelayL32 : Delay  DelayLength=1  InitialCondition=0  InputProcessing=Columns as channels (frame based)
  FootSumR32 : Sum  Inputs=++|  AccumDataTypeStr=fixdt(1,30,27)  OutDataTypeStr=fixdt(1,30,27)  RndMeth=Convergent
  h(10) : Gain  Gain=-3.00782423407123057e-05  ParamDataTypeStr=fixdt(1,13,12)  OutDataTypeStr=fixdt(1,29,27)  RndMeth=Convergent
  h(11) : Gain  Gain=0.00341338244199415955  ParamDataTypeStr=fixdt(1,13,12)  OutDataTypeStr=fixdt(1,29,27)  RndMeth=Convergent
  h(12) : Gain  Gain=-0.00235549051439376154  ParamDataTypeStr=fixdt(1,13,12)  OutDataTypeStr=fixdt(1,29,27)  RndMeth=Convergent
  h(13) : Gain  Gain=-0.00359543725669746878  ParamDataTypeStr=fixdt(1,13,12)  OutDataTypeStr=fixdt(1,29,27)  RndMeth=Convergent
  h(14) : Gain  Gain=0.00596383253332515538  ParamDataTypeStr=fixdt(1,13,12)  OutDataTypeStr=fixdt(1,29,27)  RndMeth=Convergent
  h(15) : Gain  Gain=0.00118842943627842893  ParamDataTypeStr=fixdt(1,13,12)  OutDataTypeStr=fixdt(1,29,27)  RndMeth=Convergent
  h(16) : Gain  Gain=-0.00929736814227217004  ParamDataTypeStr=fixdt(1,13,12)  OutDataTypeStr=fixdt(1,29,27)  RndMeth=Convergent
  h(17) : Gain  Gain=0.00452694246563901601  ParamDataTypeStr=fixdt(1,13,12)  OutDataTypeStr=fixdt(1,29,27)  RndMeth=Convergent
  h(18) : Gain  Gain=0.00988717854237792897  ParamDataTypeStr=fixdt(1,13,12)  OutDataTypeStr=fixdt(1,29,27)  RndMeth=Convergent
  h(19) : Gain  Gain=-0.0127452568612851334  ParamDataTypeStr=fixdt(1,13,12)  OutDataTypeStr=fixdt(1,29,27)  RndMeth=Convergent
  h(2) : Gain  Gain=-2.01758730162940583e-05  ParamDataTypeStr=fixdt(1,13,12)  OutDataTypeStr=fixdt(1,29,27)  RndMeth=Convergent
  h(20) : Gain  Gain=-0.00510213588050494223  ParamDataTypeStr=fixdt(1,13,12)  OutDataTypeStr=fixdt(1,29,27)  RndMeth=Convergent
  h(21) : Gain  Gain=0.0207062988382947788  ParamDataTypeStr=fixdt(1,13,12)  OutDataTypeStr=fixdt(1,29,27)  RndMeth=Convergent
  h(22) : Gain  Gain=-0.0066978423095265362  ParamDataTypeStr=fixdt(1,13,12)  OutDataTypeStr=fixdt(1,29,27)  RndMeth=Convergent
  h(23) : Gain  Gain=-0.0238959299794105767  ParamDataTypeStr=fixdt(1,13,12)  OutDataTypeStr=fixdt(1,29,27)  RndMeth=Convergent
  h(24) : Gain  Gain=0.0251447336934165142  ParamDataTypeStr=fixdt(1,13,12)  OutDataTypeStr=fixdt(1,29,27)  RndMeth=Convergent
  h(25) : Gain  Gain=0.0166287639766018736  ParamDataTypeStr=fixdt(1,13,12)  OutDataTypeStr=fixdt(1,29,27)  RndMeth=Convergent
  h(26) : Gain  Gain=-0.0474781320609944518  ParamDataTypeStr=fixdt(1,13,12)  OutDataTypeStr=fixdt(1,29,27)  RndMeth=Convergent
  h(27) : Gain  Gain=0.00829237505996927547  ParamDataTypeStr=fixdt(1,13,12)  OutDataTypeStr=fixdt(1,29,27)  RndMeth=Convergent
  h(28) : Gain  Gain=0.0690683880945900525  ParamDataTypeStr=fixdt(1,13,12)  OutDataTypeStr=fixdt(1,29,27)  RndMeth=Convergent
  h(29) : Gain  Gain=-0.0673387281007992167  ParamDataTypeStr=fixdt(1,13,12)  OutDataTypeStr=fixdt(1,29,27)  RndMeth=Convergent
  h(3) : Gain  Gain=-4.78076866566590479e-05  ParamDataTypeStr=fixdt(1,13,12)  OutDataTypeStr=fixdt(1,29,27)  RndMeth=Convergent
  h(30) : Gain  Gain=-0.0847467581519047164  ParamDataTypeStr=fixdt(1,13,12)  OutDataTypeStr=fixdt(1,29,27)  RndMeth=Convergent
  h(31) : Gain  Gain=0.302631264758983887  ParamDataTypeStr=fixdt(1,13,12)  OutDataTypeStr=fixdt(1,29,27)  RndMeth=Convergent
  h(32) : Gain  Gain=0.587266701839317617  ParamDataTypeStr=fixdt(1,13,12)  OutDataTypeStr=fixdt(1,29,27)  RndMeth=Convergent
  h(4) : Gain  Gain=0.000255835524546673776  ParamDataTypeStr=fixdt(1,13,12)  OutDataTypeStr=fixdt(1,29,27)  RndMeth=Convergent
  h(5) : Gain  Gain=-6.13227082388768404e-05  ParamDataTypeStr=fixdt(1,13,12)  OutDataTypeStr=fixdt(1,29,27)  RndMeth=Convergent
  h(6) : Gain  Gain=-0.000699154133393691934  ParamDataTypeStr=fixdt(1,13,12)  OutDataTypeStr=fixdt(1,29,27)  RndMeth=Convergent
  h(7) : Gain  Gain=0.000731870801887882618  ParamDataTypeStr=fixdt(1,13,12)  OutDataTypeStr=fixdt(1,29,27)  RndMeth=Convergent
  h(8) : Gain  Gain=0.000875027992170180876  ParamDataTypeStr=fixdt(1,13,12)  OutDataTypeStr=fixdt(1,29,27)  RndMeth=Convergent
  h(9) : Gain  Gain=-0.00204490131022380325  ParamDataTypeStr=fixdt(1,13,12)  OutDataTypeStr=fixdt(1,29,27)  RndMeth=Convergent
  Output : Outport
  wires:
  Input/1 -> ConvertIn/1
  ConvertIn/1 -> BodyDelayL2/1
  BodyDelayL2/1 -> BodySumL2/1, BodyDelayL3/1
  BodySumL2/1 -> h(2)/1
  h(2)/1 -> BodySumR3/2
  BodyDelayR2/1 -> BodySumL2/2
  BodyDelayL3/1 -> BodySumL3/1, BodyDelayL4/1
  BodySumL3/1 -> h(3)/1
  h(3)/1 -> BodySumR3/1
  BodyDelayR3/1 -> BodySumL3/2, BodyDelayR2/1
  BodySumR3/1 -> BodySumR4/2
  BodyDelayL4/1 -> BodySumL4/1, BodyDelayL5/1
  BodySumL4/1 -> h(4)/1
  h(4)/1 -> BodySumR4/1
  BodyDelayR4/1 -> BodySumL4/2, BodyDelayR3/1
  BodySumR4/1 -> BodySumR5/2
  BodyDelayL5/1 -> BodySumL5/1, BodyDelayL6/1
  BodySumL5/1 -> h(5)/1
  h(5)/1 -> BodySumR5/1
  BodyDelayR5/1 -> BodySumL5/2, BodyDelayR4/1
  BodySumR5/1 -> BodySumR6/2
  BodyDelayL6/1 -> BodySumL6/1, BodyDelayL7/1
  BodySumL6/1 -> h(6)/1
  h(6)/1 -> BodySumR6/1
  BodyDelayR6/1 -> BodySumL6/2, BodyDelayR5/1
  BodySumR6/1 -> BodySumR7/2
  BodyDelayL7/1 -> BodySumL7/1, BodyDelayL8/1
  BodySumL7/1 -> h(7)/1
  h(7)/1 -> BodySumR7/1
  BodyDelayR7/1 -> BodySumL7/2, BodyDelayR6/1
  BodySumR7/1 -> BodySumR8/2
  BodyDelayL8/1 -> BodySumL8/1, BodyDelayL9/1
  BodySumL8/1 -> h(8)/1
  h(8)/1 -> BodySumR8/1
  BodyDelayR8/1 -> BodySumL8/2, BodyDelayR7/1
  BodySumR8/1 -> BodySumR9/2
  BodyDelayL9/1 -> BodySumL9/1, BodyDelayL10/1
  BodySumL9/1 -> h(9)/1
  h(9)/1 -> BodySumR9/1
  BodyDelayR9/1 -> BodySumL9/2, BodyDelayR8/1
  BodySumR9/1 -> BodySumR10/2
  BodyDelayL10/1 -> BodySumL10/1, BodyDelayL11/1
  BodySumL10/1 -> h(10)/1
  h(10)/1 -> BodySumR10/1
  BodyDelayR10/1 -> BodySumL10/2, BodyDelayR9/1
  BodySumR10/1 -> BodySumR11/2
  BodyDelayL11/1 -> BodySumL11/1, BodyDelayL12/1
  BodySumL11/1 -> h(11)/1
  h(11)/1 -> BodySumR11/1
  BodyDelayR11/1 -> BodySumL11/2, BodyDelayR10/1
  BodySumR11/1 -> BodySumR12/2
  BodyDelayL12/1 -> BodySumL12/1, BodyDelayL13/1
  BodySumL12/1 -> h(12)/1
  h(12)/1 -> BodySumR12/1
  BodyDelayR12/1 -> BodySumL12/2, BodyDelayR11/1
  BodySumR12/1 -> BodySumR13/2
  BodyDelayL13/1 -> BodySumL13/1, BodyDelayL14/1
  BodySumL13/1 -> h(13)/1
  h(13)/1 -> BodySumR13/1
  BodyDelayR13/1 -> BodySumL13/2, BodyDelayR12/1
  BodySumR13/1 -> BodySumR14/2
  BodyDelayL14/1 -> BodySumL14/1, BodyDelayL15/1
  BodySumL14/1 -> h(14)/1
  h(14)/1 -> BodySumR14/1
  BodyDelayR14/1 -> BodySumL14/2, BodyDelayR13/1
  BodySumR14/1 -> BodySumR15/2
  BodyDelayL15/1 -> BodySumL15/1, BodyDelayL16/1
  BodySumL15/1 -> h(15)/1
  h(15)/1 -> BodySumR15/1
  BodyDelayR15/1 -> BodySumL15/2, BodyDelayR14/1
  BodySumR15/1 -> BodySumR16/2
  BodyDelayL16/1 -> BodySumL16/1, BodyDelayL17/1
  BodySumL16/1 -> h(16)/1
  h(16)/1 -> BodySumR16/1
  BodyDelayR16/1 -> BodySumL16/2, BodyDelayR15/1
  BodySumR16/1 -> BodySumR17/2
  BodyDelayL17/1 -> BodySumL17/1, BodyDelayL18/1
  BodySumL17/1 -> h(17)/1
  h(17)/1 -> BodySumR17/1
  BodyDelayR17/1 -> BodySumL17/2, BodyDelayR16/1
  BodySumR17/1 -> BodySumR18/2
  BodyDelayL18/1 -> BodySumL18/1, BodyDelayL19/1
  BodySumL18/1 -> h(18)/1
  h(18)/1 -> BodySumR18/1
  BodyDelayR18/1 -> BodySumL18/2, BodyDelayR17/1
  BodySumR18/1 -> BodySumR19/2
  BodyDelayL19/1 -> BodySumL19/1, BodyDelayL20/1
  BodySumL19/1 -> h(19)/1
  h(19)/1 -> BodySumR19/1
  BodyDelayR19/1 -> BodySumL19/2, BodyDelayR18/1
  BodySumR19/1 -> BodySumR20/2
  BodyDelayL20/1 -> BodySumL20/1, BodyDelayL21/1
  BodySumL20/1 -> h(20)/1
  h(20)/1 -> BodySumR20/1
  BodyDelayR20/1 -> BodySumL20/2, BodyDelayR19/1
  BodySumR20/1 -> BodySumR21/2
  BodyDelayL21/1 -> BodySumL21/1, BodyDelayL22/1
  BodySumL21/1 -> h(21)/1
  h(21)/1 -> BodySumR21/1
  BodyDelayR21/1 -> BodySumL21/2, BodyDelayR20/1
  BodySumR21/1 -> BodySumR22/2
  BodyDelayL22/1 -> BodySumL22/1, BodyDelayL23/1
  BodySumL22/1 -> h(22)/1
  h(22)/1 -> BodySumR22/1
  BodyDelayR22/1 -> BodySumL22/2, BodyDelayR21/1
  BodySumR22/1 -> BodySumR23/2
  BodyDelayL23/1 -> BodySumL23/1, BodyDelayL24/1
  BodySumL23/1 -> h(23)/1
  h(23)/1 -> BodySumR23/1
  BodyDelayR23/1 -> BodySumL23/2, BodyDelayR22/1
  BodySumR23/1 -> BodySumR24/2
  BodyDelayL24/1 -> BodySumL24/1, BodyDelayL25/1
  BodySumL24/1 -> h(24)/1
  h(24)/1 -> BodySumR24/1
  BodyDelayR24/1 -> BodySumL24/2, BodyDelayR23/1
  BodySumR24/1 -> BodySumR25/2
  BodyDelayL25/1 -> BodySumL25/1, BodyDelayL26/1
  BodySumL25/1 -> h(25)/1
  h(25)/1 -> BodySumR25/1
  BodyDelayR25/1 -> BodySumL25/2, BodyDelayR24/1
  BodySumR25/1 -> BodySumR26/2
  BodyDelayL26/1 -> BodySumL26/1, BodyDelayL27/1
  BodySumL26/1 -> h(26)/1
  h(26)/1 -> BodySumR26/1
  BodyDelayR26/1 -> BodySumL26/2, BodyDelayR25/1
  BodySumR26/1 -> BodySumR27/2
  BodyDelayL27/1 -> BodySumL27/1, BodyDelayL28/1
  BodySumL27/1 -> h(27)/1
  h(27)/1 -> BodySumR27/1
  BodyDelayR27/1 -> BodySumL27/2, BodyDelayR26/1
  BodySumR27/1 -> BodySumR28/2
  BodyDelayL28/1 -> BodySumL28/1, BodyDelayL29/1
  BodySumL28/1 -> h(28)/1
  h(28)/1 -> BodySumR28/1
  BodyDelayR28/1 -> BodySumL28/2, BodyDelayR27/1
  BodySumR28/1 -> BodySumR29/2
  BodyDelayL29/1 -> BodySumL29/1, BodyDelayL30/1
  BodySumL29/1 -> h(29)/1
  h(29)/1 -> BodySumR29/1
  BodyDelayR29/1 -> BodySumL29/2, BodyDelayR28/1
  BodySumR29/1 -> BodySumR30/2
  BodyDelayL30/1 -> BodySumL30/1, BodyDelayL31/1
  BodySumL30/1 -> h(30)/1
  h(30)/1 -> BodySumR30/1
  BodyDelayR30/1 -> BodySumL30/2, BodyDelayR29/1
  BodySumR30/1 -> BodySumR31/2
  BodyDelayL31/1 -> BodySumL31/1, FootDelayL32/1
  BodySumL31/1 -> h(31)/1
  h(31)/1 -> BodySumR31/1
  BodyDelayR31/1 -> BodySumL31/2, BodyDelayR30/1
  BodySumR31/1 -> FootSumR32/2
  FootDelayL32/1 -> h(32)/1, BodyDelayR31/1
  h(32)/1 -> FootSumR32/1
  FootSumR32/1 -> ConvertOut/1
  ConvertOut/1 -> Output/1
